simulink library "find6DOF_cl"  (R2018b)
settings: Solver=VariableStepAuto  StartTime=0.0  StopTime=10.0  RelTol=1e-3
values from neighbouring files (symbols this model uses):
  GFC2Bottom = calculateRotationMatrix(botEulerAngles(1),botEulerAngles(2),botEulerAngles(3))    [find6DOF_init.m]
  GFC2Side = calculateRotationMatrix(sideEulerAngles(1),sideEulerAngles(2),sideEulerAngles(3))    [find6DOF_init.m]
  GFC2Slant = calculateRotationMatrix(slantEulerAngles(1),slantEulerAngles(2),slantEulerAngles(3))    [find6DOF_init.m]
libraries: FindUnitVectorComponents_ul x4, findEulerAngles_ul x1, findPosition_ul x1, findUnitVectors_ul x1
settings Model: Creator=mcobb  LastModifiedBy=mae-ncsucore

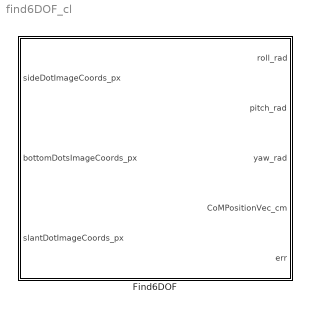
== system find6DOF_cl ==
  Find6DOF : Subsystem  mask{imageDims_px=[1080 2048], initialCoMPositionVec_cm=[0 0 50], cameraFOVAngles_deg=[30 30], sideEulerAngles=[-90 90 0], sideCamPositionVec_cm=[0 0 40], botEulerAngles=[0 0 180], botCamPositionVec_cm=[0 0 0], slantEulerAngles=[180 130 0], slantCamPositionVec_cm=[-20 0 0], sideSeparation_cm=2, sidePositionVecBF_cm=[1 1 1], bottomASeparation_cm=2, botAPositionVecBF_cm=[1 1 1], bottomBSeparation_cm=2, botBPositionVecBG_cm=[1 1 1]}
      mask prompts: imageDims_px "Image Dimensions [rows, cols] [px]"; initialCoMPositionVec_cm "Initial CoM Position Vector [cm]"; cameraFOVAngles_deg "Field of View Angles [horiz, vert] [deg]"; sideEulerAngles "Euler Angles [roll pitch yaw] [deg]"; sideCamPositionVec_cm "Position Vector [cm]"; botEulerAngles "Euler Angles [roll pitch yaw]  [deg]"; botCamPositionVec_cm "Position Vector [cm]"; slantEulerAngles "Euler Angles [roll pitch yaw]  [deg]"; slantCamPositionVec_cm "Position Vec [cm]"; sideSeparation_cm "Separation Distance [cm]"; sidePositionVecBF_cm "Centroid Position in Body Frame [cm]"; bottomASeparation_cm "Separation Distance [cm]"; botAPositionVecBF_cm "Centroid Position in Body Frame [cm]"; bottomBSeparation_cm "Separation Distance [cm]"; botBPositionVecBG_cm "Centroid Position in Body Frame [cm]"
      mask init:
      | find6DOF_init
      mask DialogControl Container4 Prompt: Camera Properties
      mask DialogControl Container14 Prompt: Side Camera
      mask DialogControl Container17 Prompt: Bottom Camera
      mask DialogControl Container18 Prompt: Slant Camera
      mask DialogControl Container13 Prompt: Dot Properties
      mask DialogControl Container11 Prompt: Side Dots
      mask DialogControl Container12 Prompt: Bottom Dot Set A
      mask DialogControl Container15 Prompt: Bottom Dot Set B
      mask Display:
      | image('blockImage.png',[.2, .2, .6, .6],'on');
      | 
      | port_label('input',1,'Side')
      | port_label('input',2,'Bottom')
      | port_label('input',3,'Slant')
      | 
      | port_label('output',1,'roll_rad')
      | port_label('output',2,'pitch_rad')
      | port_label('output',3,'yaw_rad')
      | port_label('output',4,'CoMPosVec_cm')
      | port_label('output',5,'err')
      | 
      | text(0.5, 1, 'Resolve 6 DOF', 'horizontalAlignment', 'center', ...
      |   'verticalAlignment', 'top')

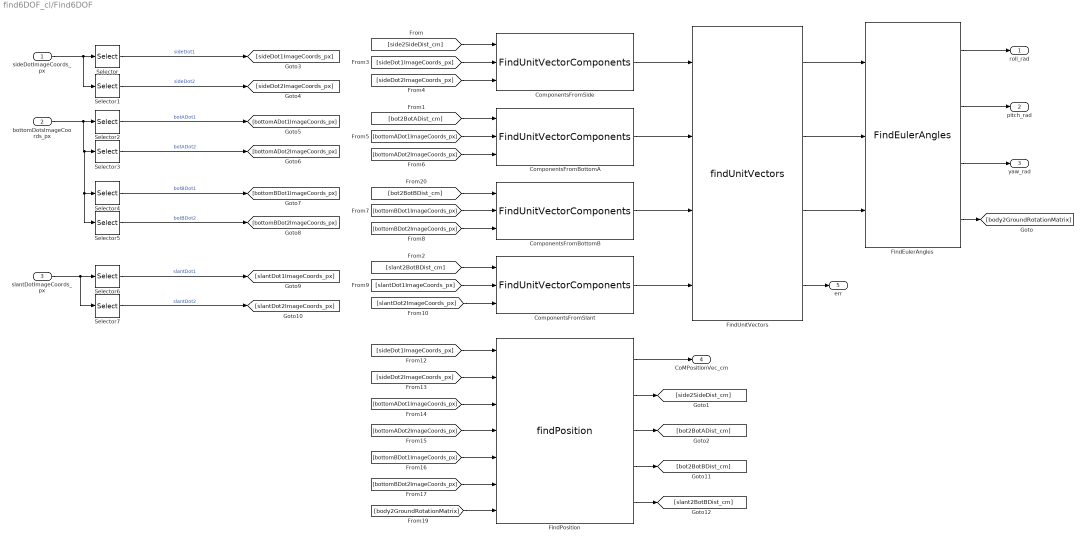
== system find6DOF_cl/Find6DOF ==
  sideDotImageCoords_px : Inport
  bottomDotsImageCoords_px : Inport  Port=2
  slantDotImageCoords_px : Inport  Port=3
  ComponentsFromBottomA : FindUnitVectorComponents_ul/FindUnitVectorComponents  cameraViewAngleVec_deg=cameraFOVAngles_deg  cam2GroundRotationMatrix=GFC2Bottom'  imageDimensions=imageDims_px
  ComponentsFromBottomB : FindUnitVectorComponents_ul/FindUnitVectorComponents  cameraViewAngleVec_deg=cameraFOVAngles_deg  cam2GroundRotationMatrix=GFC2Bottom'  imageDimensions=imageDims_px
  ComponentsFromSide : FindUnitVectorComponents_ul/FindUnitVectorComponents  cameraViewAngleVec_deg=cameraFOVAngles_deg  cam2GroundRotationMatrix=GFC2Side'  imageDimensions=imageDims_px
  ComponentsFromSlant : FindUnitVectorComponents_ul/FindUnitVectorComponents  cameraViewAngleVec_deg=cameraFOVAngles_deg  cam2GroundRotationMatrix=GFC2Slant'  imageDimensions=imageDims_px
  FindEulerAngles : findEulerAngles_ul/FindEulerAngles  SystemSampleTime=-1
  FindPosition : findPosition_ul/findPosition  sideCameraPositionVec_cm=sideCamPositionVec_cm  bottomCameraPositionVec_cm=botCamPositionVec_cm  slantCameraPositionVec_cm=slantCamPositionVec_cm  sideDotPositionVec_cm=sidePositionVecBF_cm  bottomDotAPositionVec_cm=botAPositionVecBF_cm  bottomDotBPositionVec_cm=botBPositionVecBG_cm  side2GroundRotationMatrix=GFC2Side'  bot2GroundRotationMatrix=GFC2Bottom'  slant2GroundRotationMatrix=GFC2Slant'  initialCoMPositionVec_cm=initialCoMPositionVec_cm  imageDims=imageDims_px  cameraFOVAngle_deg=cameraFOVAngles_deg
  FindUnitVectors : findUnitVectors_ul/findUnitVectors  sideSeparation_cm=sideSeparation_cm  bottomASeparation_cm=bottomASeparation_cm  bottomBSeparation_cm=bottomBSeparation_cm  DSB=DSB  DBL=DBL
  Selector : Selector  InputPortWidth=4  IndexOptions=Index vector (dialog)  Indices=[1 2]  OutputSizes=1
  Selector1 : Selector  InputPortWidth=4  IndexOptions=Index vector (dialog)  Indices=[3 4]  OutputSizes=1
  Selector2 : Selector  InputPortWidth=8  IndexOptions=Index vector (dialog)  Indices=[1 2]  OutputSizes=1
  Selector3 : Selector  InputPortWidth=8  IndexOptions=Index vector (dialog)  Indices=[3 4]  OutputSizes=1
  Selector4 : Selector  InputPortWidth=8  IndexOptions=Index vector (dialog)  Indices=[5 6]  OutputSizes=1
  Selector5 : Selector  InputPortWidth=8  IndexOptions=Index vector (dialog)  Indices=[7 8]  OutputSizes=1
  Selector6 : Selector  InputPortWidth=4  IndexOptions=Index vector (dialog)  Indices=[1 2]  OutputSizes=1
  Selector7 : Selector  InputPortWidth=4  IndexOptions=Index vector (dialog)  Indices=[3 4]  OutputSizes=1
  roll_rad : Outport  Unit=rad
  pitch_rad : Outport  Port=2  Unit=rad
  yaw_rad : Outport  Port=3  Unit=rad
  CoMPositionVec_cm : Outport  Port=4  Unit=cm
  err : Outport  Port=5
  wires:
  ComponentsFromSide/1 -> FindUnitVectors/1
  ComponentsFromBottomA/1 -> FindUnitVectors/2
  ComponentsFromBottomB/1 -> FindUnitVectors/3
  ComponentsFromSlant/1 -> FindUnitVectors/4
  FindUnitVectors/2 -> FindEulerAngles/2
  FindUnitVectors/1 -> FindEulerAngles/1
  FindUnitVectors/3 -> FindEulerAngles/3
  FindPosition/1 -> CoMPositionVec_cm/1
  [sideDot1ImageCoords_px] -> ComponentsFromSide/2
  [sideDot2ImageCoords_px] -> ComponentsFromSide/3
  [bottomADot1ImageCoords_px] -> ComponentsFromBottomA/2
  [bottomADot2ImageCoords_px] -> ComponentsFromBottomA/3
  [bottomBDot1ImageCoords_px] -> ComponentsFromBottomB/2
  [bottomBDot2ImageCoords_px] -> ComponentsFromBottomB/3
  [slantDot1ImageCoords_px] -> ComponentsFromSlant/2
  [slantDot2ImageCoords_px] -> ComponentsFromSlant/3
  FindEulerAngles/1 -> roll_rad/1
  FindEulerAngles/2 -> pitch_rad/1
  FindEulerAngles/3 -> yaw_rad/1
  FindEulerAngles/4 -> [body2GroundRotationMatrix]
  FindUnitVectors/4 -> err/1
  FindPosition/2 -> [side2SideDist_cm]
  FindPosition/3 -> [bot2BotADist_cm]
  FindPosition/5 -> [slant2BotBDist_cm]
  FindPosition/4 -> [bot2BotBDist_cm]
  [side2SideDist_cm] -> ComponentsFromSide/1
  [bot2BotADist_cm] -> ComponentsFromBottomA/1
  [slant2BotBDist_cm] -> ComponentsFromSlant/1
  [bot2BotBDist_cm] -> ComponentsFromBottomB/1
  Selector/1 -> [sideDot1ImageCoords_px]  "sideDot1"
  Selector1/1 -> [sideDot2ImageCoords_px]  "sideDot2"
  sideDotImageCoords_px/1 -> Selector1/1, Selector/1
  bottomDotsImageCoords_px/1 -> Selector5/1, Selector4/1, Selector3/1, Selector2/1
  Selector2/1 -> [bottomADot1ImageCoords_px]  "botADot1"
  Selector3/1 -> [bottomADot2ImageCoords_px]  "botADot2"
  Selector4/1 -> [bottomBDot1ImageCoords_px]  "botBDot1"
  Selector5/1 -> [bottomBDot2ImageCoords_px]  "botBDot2"
  Selector6/1 -> [slantDot1ImageCoords_px]  "slantDot1"
  slantDotImageCoords_px/1 -> Selector7/1, Selector6/1
  Selector7/1 -> [slantDot2ImageCoords_px]  "slantDot2"
  [sideDot1ImageCoords_px] -> FindPosition/1
  [sideDot2ImageCoords_px] -> FindPosition/2
  [bottomADot1ImageCoords_px] -> FindPosition/3
  [bottomADot2ImageCoords_px] -> FindPosition/4
  [bottomBDot1ImageCoords_px] -> FindPosition/5
  [bottomBDot2ImageCoords_px] -> FindPosition/6
  [body2GroundRotationMatrix] -> FindPosition/7
